simulink model "ad_logic_analyzer"  (R2015b)
settings: Solver=ode45  StartTime=0.0  StopTime=10.0  RelTol=1e-3
StopFcn:
  | edit ad_view_logic
  | ad_view_logic
libraries: simulink x2
settings Model: Creator=amatsumo  LastModifiedBy=amatsumo
settings DataIOCC: SaveFormat=Array
settings DebuggingCC: UnderspecifiedInitializationDetection=Classic  MergeDetectMultiDrivingBlocksExec=none  SolverPrmCheckMsg=warning  StateNameClashWarn=warning
settings HardwareCC: ProdBitPerPointer=32  ProdLargestAtomicFloat=None  ProdIntDivRoundTo=Undefined  ProdEndianess=Unspecified  ProdWordSize=32  ProdHWDeviceType=32-bit Generic
settings GRTTargetCC: GeneratePreprocessorConditionals=Disable all
settings ConfigComp: CovModelRefEnable=Off  CovSFcnEnable=off

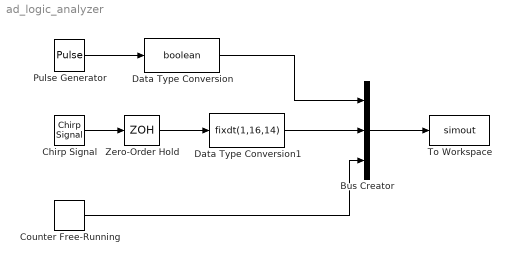
== system ad_logic_analyzer ==
  Bus Creator : BusCreator  Inputs=3
  Chirp Signal : simulink/Sources/Chirp Signal  f1=10  T=10  f2=500
  Counter Free-Running : simulink/Sources/Counter Free-Running  NumBits=16  tsamp=1/1000
  Data Type Conversion : DataTypeConversion  OutDataTypeStr=boolean
  Data Type Conversion1 : DataTypeConversion  OutDataTypeStr=fixdt(1,16,14)
  Pulse Generator : DiscretePulseGenerator  SampleTime=1/1000
  To Workspace : ToWorkspace  VariableName=simout  SaveFormat=Timeseries  SampleTime=-1
  Zero-Order Hold : ZeroOrderHold  SampleTime=1/1000
  wires:
  Chirp Signal/1 -> Zero-Order Hold/1
  Pulse Generator/1 -> Data Type Conversion/1
  Zero-Order Hold/1 -> Data Type Conversion1/1
  Data Type Conversion/1 -> Bus Creator/1
  Data Type Conversion1/1 -> Bus Creator/2
  Counter Free-Running/1 -> Bus Creator/3
  Bus Creator/1 -> To Workspace/1
